simulink model "ACC1"  (R2018b)
settings: Solver=FixedStepAuto  StartTime=0.0  StopTime=inf  RelTol=1e-3  EnableMultiTasking=on
libraries: arduinolib x5, LCDlib x1, arduinosensorlib x1
settings Model: SimulationMode=external  ExtModeTrigDuration=2  Creator=Pruthvi Gabani  LastModifiedBy=singh
settings OptimizationCC: EnhancedBackFolding=on  PassReuseOutputArgsThreshold=0  MaxStackSize=64  OptimizeBlockOrder=speed  DifferentSizesBufferReuse=on  OptimizationCustomize=off
settings DebuggingCC: ParameterTunabilityLossMsg=error
settings HardwareCC: ProdBitPerInt=16  ProdBitPerPointer=16  ProdBitPerSizeT=16  ProdBitPerPtrDiffT=16  ProdLargestAtomicFloat=None  ProdWordSize=8  ProdHWDeviceType=Atmel->AVR
settings SFSimCC: MATLABDynamicMemAlloc=off
settings RTWCC: SystemTargetFile=ert.tlc  HardwareBoard=Arduino Uno  TemplateMakefile=ert_default_tmf  GenerateReport=on  Toolchain=Arduino AVR  BuildConfiguration=Faster Runs  LaunchReport=on
settings CodeAppCC: ForceParamTrailComments=on  OperatorAnnotations=on
settings ERTTargetCC: ERTCustomFileBanners=off  SupportContinuousTime=on  SupportNonInlinedSFcns=on  RemoveResetFunc=off  SupportVariableSizeSignals=on  ModelStepFunctionPrototypeControlCompliant=off

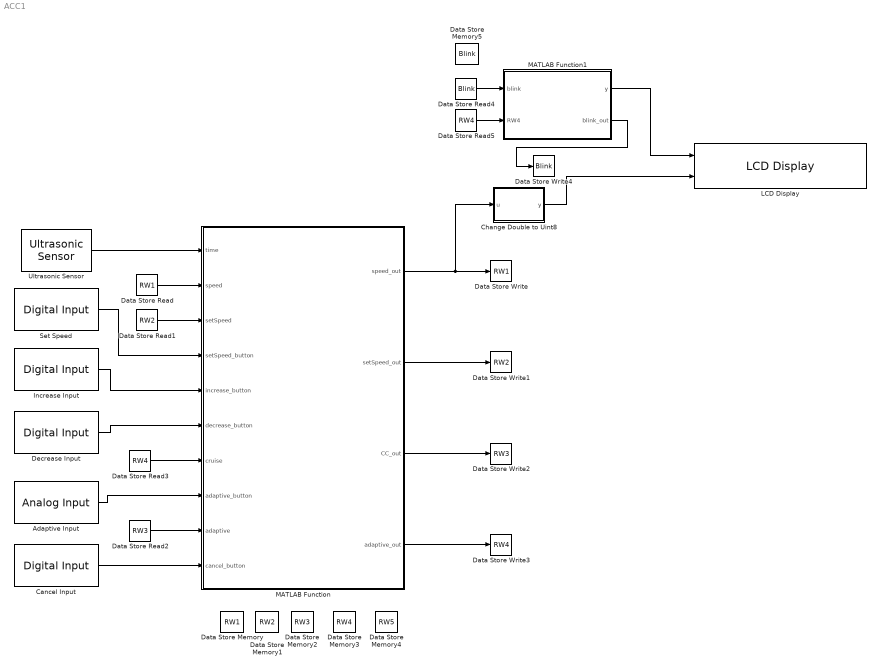
== system ACC1 ==
  Adaptive Input : arduinolib/Analog Input  pinNumber=3  ReadResultsOnly=off  ConversionTriggerSource=Software  ExternalTriggerType=uint32(0)  OutputDataType=uint16  EnableConversionCompleteNotify=off  EnableOuputStatus=off  SampleTime=1  blockPlatform=arduino
  Cancel Input : arduinolib/Digital Input  pinNumber=6  SampleTime=1  blockPlatform=arduino
      settings: SourceProductName=Simulink Support Package for Arduino Hardware
  Change Double to Uint8 : MATLAB Function  TreatAsAtomicUnit=on
  Data Store Memory : DataStoreMemory  DataStoreName=RW1  ReadBeforeWriteMsg=warning  WriteAfterWriteMsg=warning  WriteAfterReadMsg=warning  ShowAdditionalParam=off
  Data Store Memory1 : DataStoreMemory  DataStoreName=RW2  ReadBeforeWriteMsg=warning  WriteAfterWriteMsg=warning  WriteAfterReadMsg=warning  ShowAdditionalParam=off
  Data Store Memory2 : DataStoreMemory  DataStoreName=RW3  ReadBeforeWriteMsg=warning  WriteAfterWriteMsg=warning  WriteAfterReadMsg=warning  ShowAdditionalParam=off
  Data Store Memory3 : DataStoreMemory  DataStoreName=RW4  ReadBeforeWriteMsg=warning  WriteAfterWriteMsg=warning  WriteAfterReadMsg=warning  ShowAdditionalParam=off
  Data Store Memory4 : DataStoreMemory  DataStoreName=RW5  ReadBeforeWriteMsg=warning  WriteAfterWriteMsg=warning  WriteAfterReadMsg=warning  ShowAdditionalParam=off
  Data Store Memory5 : DataStoreMemory  DataStoreName=Blink  ReadBeforeWriteMsg=warning  WriteAfterWriteMsg=warning  WriteAfterReadMsg=warning  ShowAdditionalParam=off
  Data Store Read : DataStoreRead  DataStoreName=RW1
  Data Store Read1 : DataStoreRead  DataStoreName=RW2
  Data Store Read2 : DataStoreRead  DataStoreName=RW3
  Data Store Read3 : DataStoreRead  DataStoreName=RW4
  Data Store Read4 : DataStoreRead  DataStoreName=Blink
  Data Store Read5 : DataStoreRead  DataStoreName=RW4
  Data Store Write : DataStoreWrite  DataStoreName=RW1
  Data Store Write1 : DataStoreWrite  DataStoreName=RW2
  Data Store Write2 : DataStoreWrite  DataStoreName=RW3
  Data Store Write3 : DataStoreWrite  DataStoreName=RW4
  Data Store Write4 : DataStoreWrite  DataStoreName=Blink
  Decrease Input : arduinolib/Digital Input  pinNumber=8  SampleTime=1  blockPlatform=arduino
      settings: SourceProductName=Simulink Support Package for Arduino Hardware
  Increase Input : arduinolib/Digital Input  pinNumber=13  SampleTime=1  blockPlatform=arduino
      settings: SourceProductName=Simulink Support Package for Arduino Hardware
  LCD Display : LCDlib/LCD Display  pins=[12,11,5,4,3,2]
      settings: SourceProductName=LCD Library
  MATLAB Function : MATLAB Function  TreatAsAtomicUnit=on
  MATLAB Function1 : MATLAB Function  TreatAsAtomicUnit=on
  Set Speed : arduinolib/Digital Input  pinNumber=7  SampleTime=1  blockPlatform=arduino
      settings: SourceProductName=Simulink Support Package for Arduino Hardware
  Ultrasonic Sensor : arduinosensorlib/Ultrasonic Sensor  NumSignalPins=2  TrigPin=9  EchoPin=10  SignalPin=3  SampleTime_=1  blockPlatform=ARDUINO
      settings: SourceProductName=Simulink Support Package for Arduino Hardware
  wires:
  Cancel Input/1 -> MATLAB Function/10(cancel_button)
  Adaptive Input/1 -> MATLAB Function/8(adaptive_button)
  Decrease Input/1 -> MATLAB Function/6(decrease_button)
  Set Speed/1 -> MATLAB Function/4(setSpeed_button)
  Increase Input/1 -> MATLAB Function/5(increase_button)
  Change Double to Uint8/1(y) -> LCD Display/2
  MATLAB Function/1(speed_out) -> Change Double to Uint8/1(u), Data Store Write/1
  Ultrasonic Sensor/1 -> MATLAB Function/1(time)
  Data Store Read/1 -> MATLAB Function/2(speed)
  Data Store Read1/1 -> MATLAB Function/3(setSpeed)
  Data Store Read3/1 -> MATLAB Function/7(cruise)
  MATLAB Function/2(setSpeed_out) -> Data Store Write1/1
  MATLAB Function/3(CC_out) -> Data Store Write2/1
  MATLAB Function/4(adaptive_out) -> Data Store Write3/1
  Data Store Read2/1 -> MATLAB Function/9(adaptive)
  Data Store Read4/1 -> MATLAB Function1/1(blink)
  Data Store Read5/1 -> MATLAB Function1/2(RW4)
  MATLAB Function1/2(blink_out) -> Data Store Write4/1
  MATLAB Function1/1(y) -> LCD Display/1

== matlab function ACC1/Change Double to Uint8 ==
  data: u input; y output
function y = DouToUint8(u)
switch u
    case 0
        y = [[48],[48]];
    case 1
        y = [[48],[49]];
    case 2 
        y = [[48],[50]];
    case 3
        y = [[48],[51]];
    case 4
        y = [[48],[52]];
    case 5
        y = [[48],[53]];
    case 6
        y = [[48],[54]];
    case 7
        y = [[48],[55]];
    case 8
        y = [[48],[56]];
    case 9
        y = [[48],[57]];
    case 10
        y = [[49],[48]];
    case 11 
        y = [[49],[49]];
    case 12
        y = [[49],[50]];
    case 13
        y = [[49],[51]];
    case 14
        y = [[49],[52]];
    case 15
        y = [[49],[53]];
    case 16
        y = [[49],[54]];
    case 17
        y = [[49],[55]];
    case 18
        y = [[49],[56]];
    case 19
        y = [[49],[57]];
    case 20
        y = [[50],[48]];
    case 21 
        y = [[50],[49]];
    case 22
        y = [[50],[50]];
    case 23
        y = [[50],[51]];
    case 24
        y = [[50],[52]];
    case 25
        y = [[50],[53]];
    case 26
        y = [[50],[54]];
    case 27
        y = [[50],[55]];
    case 28
        y = [[50],[56]];
    case 29
        y = [[50],[57]];
    case 30
        y = [[51],[48]];
    case 31 
        y = [[51],[49]];
    case 32
        y = [[51],[50]];
    case 33
        y = [[51],[51]];
    case 34
        y = [[51],[52]];
    case 35
        y = [[51],[53]];
    case 36
        y = [[51],[54]];
    case 37
        y = [[51],[55]];
    case 38
        y = [[51],[56]];
    case 39
        y = [[51],[57]];
    case 40
        y = [[52],[48]];
    case 41 
        y = [[52],[49]];
    case 42
        y = [[52],[50]];
    case 43
        y = [[52],[51]];
    case 44
        y = [[52],[52]];
    case 45
        y = [[52],[53]];
    case 46
        y = [[52],[54]];
    case 47
        y = [[52],[55]];
    case 48
        y = [[52],[56]];
    case 49
        y = [[52],[57]];
    case 50
        y = [[53],[48]];
    otherwise
        y = [[48],[48]];
end

== matlab function ACC1/MATLAB Function ==
  data: time input; speed_out output; speed input; setSpeed input; setSpeed_button input; increase_button input; decrease_button input; cruise input; adaptive_button input; adaptive input; cancel_button input; setSpeed_out output; CC_out output; adaptive_out output
function [speed_out, setSpeed_out,CC_out, adaptive_out] = ACC(time,speed,setSpeed,setSpeed_button,increase_button, decrease_button,cruise,adaptive_button,adaptive,cancel_button)
    
    distance=(time*343)/2;
    
    if cancel_button
        adaptive_out=0;
        setSpeed_out=setSpeed;
        CC_out=0;
    elseif adaptive_button>800
        setSpeed_out=speed;
        adaptive_out=1;
        CC_out=0;
    elseif setSpeed_button
        setSpeed_out=speed;
        CC_out=1;
        adaptive_out=0;
    else
        setSpeed_out=setSpeed;
        CC_out=cruise;
        adaptive_out=adaptive;
    end
    
    if increase_button == 1 && ~adaptive_out == 1
        speed_out = speed+1;
    elseif decrease_button == 1 && speed>0 && ~adaptive_out == 1
        speed_out = speed-1;
    elseif CC_out ==1 
        if increase_button == 1  && ~adaptive_out == 1
            speed_out = speed+1;
        elseif decrease_button == 1 && speed>0 && ~adaptive_out == 1
            speed_out = speed-1;
        else
            speed_out = speed;
        end
    elseif adaptive_out == 1
        if (distance<20) && (speed>0)
            speed_out=speed-1;
        else
                if speed<setSpeed && distance>=20
                    speed_out= speed+1;
                else
                    speed_out=speed;
                end
        end
    else
        if speed>0
            speed_out=speed-1;
        else
            speed_out=speed;
        end
    end
end

== matlab function ACC1/MATLAB Function1 ==
  data: blink input; y output; RW4 input; blink_out output
function [y,blink_out]  = fcn(blink,RW4)

    if blink==0 && RW4
        y=[[32],[32],[32],[32],[32],[32]];
        blink_out=1;
    elseif blinkState==1 && RW4
        y=[[83],[112],[101],[101],[100],[58]]; 
        blink_out=0;
    else
        y=[[83],[112],[101],[101],[100],[58]];
        blink_out=blink;
    end
end
